simulink model "sampleModel81"  (R2021b)
settings: Solver=VariableStepAuto  StartTime=0.0  StopTime=10.0  RelTol=1e-3
undefined symbols (not defined in the file or in its folder): DiscIntNeverNeededParam
libraries: simulink x9, slpidlib x2
settings Model: Creator=user  LastModifiedBy=user

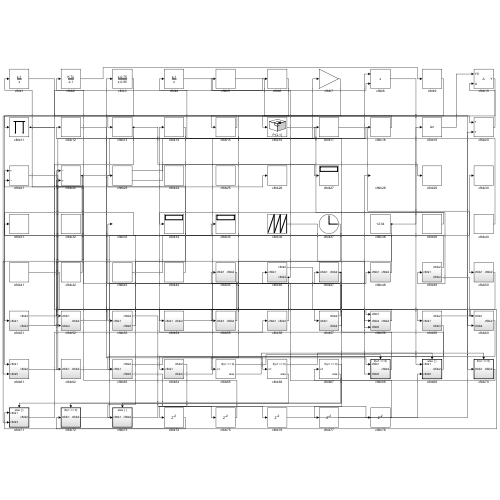
[thumbnail: Simulink's stored preview of the top-level diagram]
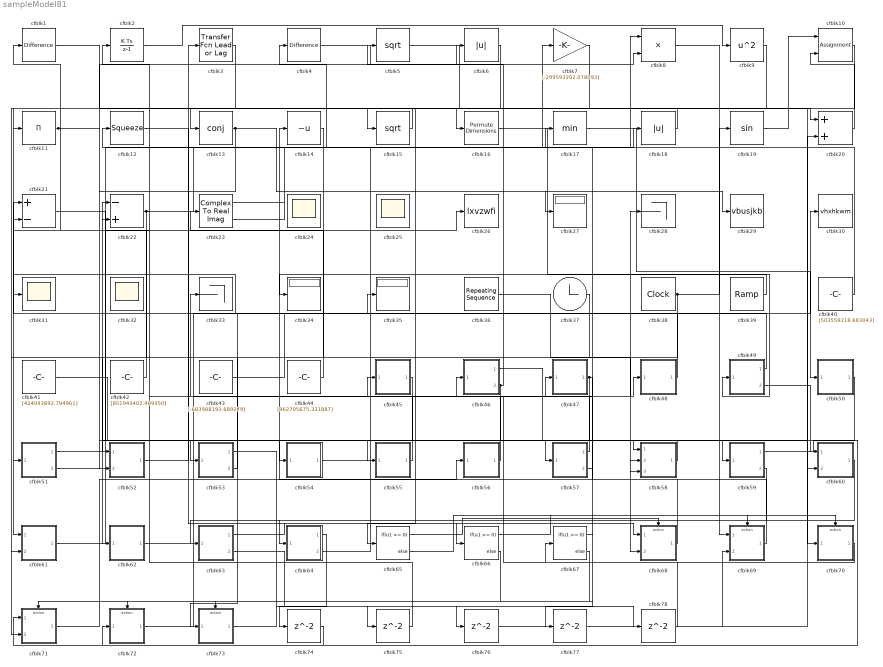
== system sampleModel81 ==
  cfblk1 : simulink/Discrete/Difference  ICPrevInput=0.0  OutMin=[]  OutMax=[]  OutDataTypeStr=Inherit: Inherit via back propagation  OutDataType=fixdt(1, 16)  OutScaling=2^-10  DoSatur=off
  cfblk10 : Assignment  DiagnosticForDimensions=Warning  IndexOptions=Index vector (dialog)  Indices=1  OutputSizes=1
  cfblk11 : Product  Inputs=*
  cfblk12 : Squeeze
  cfblk13 : Math  Operator=conj  SaturateOnIntegerOverflow=on
  cfblk14 : UnaryMinus
  cfblk15 : Sqrt  SaturateOnIntegerOverflow=on
  cfblk16 : PermuteDimensions
  cfblk17 : MinMax
  cfblk18 : Abs
  cfblk19 : Trigonometry
  cfblk2 : DiscreteIntegrator  ICPrevOutput=DiscIntNeverNeededParam  ICPrevScaledInput=DiscIntNeverNeededParam
  cfblk20 : Sum
  cfblk21 : Sum  Inputs=+-
  cfblk22 : Sum  Inputs=-+
  cfblk23 : ComplexToRealImag
  cfblk{24..25,31..32} (4 alike) : Scope
      cfblk24 settings: Floating=on
      cfblk25 settings: Floating=on
      cfblk32 settings: Floating=on
  cfblk26 : ToWorkspace  VariableName=lxvzwfi  SaveFormat=Timeseries  SampleTime=-1
  cfblk27 : Display
  cfblk28 : Terminator
  cfblk29 : ToWorkspace  VariableName=vbusjkb  SaveFormat=Timeseries  SampleTime=-1
  cfblk3 : simulink/Discrete/Transfer Fcn Lead or Lag  PoleZ=0.95  ZeroZ=0.75  ICPrevOutput=0.0  ICPrevInput=0.0  DoSatur=off
      settings: SourceProductBaseCode=SL
  cfblk30 : ToWorkspace  VariableName=vhxhkwm  SaveFormat=Timeseries  SampleTime=-1
  cfblk33 : Terminator
  cfblk34 : Display
  cfblk35 : Display
  cfblk36 : simulink/Sources/Repeating Sequence  rep_seq_t=[0 2]  rep_seq_y=[7788127.978468, 363612122.173200]
  cfblk37 : Clock
  cfblk38 : DigitalClock
  cfblk39 : simulink/Sources/Ramp  slope=[-4423.881026]  start=[41.210749]  InitialOutput=[995796.420869]
  cfblk4 : simulink/Discrete/Difference  ICPrevInput=0.0  OutMin=[]  OutMax=[]  OutDataTypeStr=Inherit: Inherit via back propagation  OutDataType=fixdt(1, 16)  OutScaling=2^-10  DoSatur=off
  cfblk40 : Constant  Value=[503559218.683043]  SampleTime=1
  cfblk41 : Constant  Value=[424093892.794961]  SampleTime=1
  cfblk42 : Constant  Value=[851943402.489350]  SampleTime=1
  cfblk43 : Constant  Value=[-683988193.689279]  SampleTime=1
  cfblk44 : Constant  Value=[962705675.331887]  SampleTime=1
  cfblk45 : Subsystem
  cfblk46 : Subsystem
  cfblk47 : Subsystem
  cfblk48 : Subsystem
  cfblk49 : Subsystem
  cfblk5 : Sqrt  SaturateOnIntegerOverflow=on
  cfblk50 : Subsystem
  cfblk51 : Subsystem
  cfblk52 : Subsystem
  cfblk53 : Subsystem
  cfblk54 : Subsystem
  cfblk55 : Subsystem
  cfblk56 : Subsystem
  cfblk57 : Subsystem
  cfblk58 : Subsystem
  cfblk59 : Subsystem
  cfblk6 : Abs
  cfblk60 : Subsystem
  cfblk61 : Subsystem
  cfblk62 : Subsystem
  cfblk63 : Subsystem
  cfblk64 : Subsystem
  cfblk65 : If  IfExpression=u1 >= 0  SampleTime=1
  cfblk66 : If  IfExpression=u1 >= 0  SampleTime=1
  cfblk67 : If  IfExpression=u1 >= 0  SampleTime=1
  cfblk68 : Subsystem  TreatAsAtomicUnit=on
  cfblk69 : Subsystem  TreatAsAtomicUnit=on
  cfblk7 : Gain  Gain=[-299593202.078093]
  cfblk70 : Subsystem  TreatAsAtomicUnit=on
  cfblk71 : Subsystem  TreatAsAtomicUnit=on
  cfblk72 : Subsystem  TreatAsAtomicUnit=on
  cfblk73 : Subsystem  TreatAsAtomicUnit=on
  cfblk{74..78} (5 alike) : Delay  SampleTime=1
  cfblk8 : Product  Inputs=**
  cfblk9 : Math  Operator=square  SaturateOnIntegerOverflow=on
  wires:
  cfblk60/1(cfblk2) -> cfblk64/1(cfblk1)
  cfblk19/1 -> cfblk10/1
  cfblk47/1(cfblk2) -> cfblk57/1(cfblk1), cfblk77/1
  cfblk69/1(cfblk2) -> cfblk47/1(cfblk1)
  cfblk57/1(cfblk2) -> cfblk33/1
  cfblk49/1(cfblk2) -> cfblk61/1(cfblk1)
  cfblk16/1 -> cfblk49/1(cfblk1)
  cfblk10/1 -> cfblk51/1(cfblk1)
  cfblk20/1 -> cfblk10/2
  cfblk17/1 -> cfblk50/1(cfblk1)
  cfblk64/2(cfblk4) -> cfblk17/1
  cfblk59/1(cfblk2) -> cfblk71/1(cfblk1)
  cfblk62/1(cfblk2) -> cfblk30/1
  cfblk71/1(cfblk2) -> cfblk56/1(cfblk1)
  cfblk68/1(cfblk2) -> cfblk14/1
  cfblk49/2(cfblk4) -> cfblk60/1(cfblk1)
  cfblk57/2(cfblk4) -> cfblk12/1
  cfblk23/1 -> cfblk27/1
  cfblk13/1 -> cfblk29/1, cfblk52/2(cfblk4)
  cfblk72/1(cfblk2) -> cfblk48/1(cfblk1)
  cfblk70/1(cfblk2) -> cfblk67/1
  cfblk39/1 -> cfblk34/1
  cfblk56/1(cfblk2) -> cfblk45/1(cfblk1)
  cfblk6/1 -> cfblk65/1
  cfblk18/1 -> cfblk13/1
  cfblk46/1(cfblk2) -> cfblk59/1(cfblk1)
  cfblk22/1 -> cfblk18/1, cfblk52/1(cfblk1), cfblk21/2
  cfblk38/1 -> cfblk19/1, cfblk55/1(cfblk1)
  cfblk63/1(cfblk2) -> cfblk68/1(cfblk1)
  cfblk12/1 -> cfblk66/1
  cfblk7/1 -> cfblk16/1
  cfblk37/1 -> cfblk71/2(cfblk3)
  cfblk59/2(cfblk3) -> cfblk63/1(cfblk1)
  cfblk21/1 -> cfblk60/2(cfblk4)
  cfblk52/1(cfblk2) -> cfblk3/1
  cfblk43/1 -> cfblk35/1
  cfblk45/1(cfblk2) -> cfblk54/1(cfblk1)
  cfblk50/1(cfblk2) -> cfblk58/1(cfblk1)
  cfblk9/1 -> cfblk15/1
  cfblk61/1(cfblk2) -> cfblk8/1
  cfblk51/1(cfblk2) -> cfblk22/1
  cfblk48/1(cfblk2) -> cfblk21/1
  cfblk58/1(cfblk2) -> cfblk53/1(cfblk1)
  cfblk11/1 -> cfblk58/2(cfblk4), cfblk6/1
  cfblk8/1 -> cfblk69/1(cfblk1)
  cfblk2/1 -> cfblk9/1
  cfblk14/1 -> cfblk73/1(cfblk1)
  cfblk54/1(cfblk2) -> cfblk28/1
  cfblk23/2 -> cfblk7/1
  cfblk41/1 -> cfblk58/3(cfblk5)
  cfblk15/1 -> cfblk11/1
  cfblk3/1 -> cfblk61/2(cfblk5)
  cfblk55/1(cfblk2) -> cfblk2/1
  cfblk36/1 -> cfblk68/2(cfblk5)
  cfblk40/1 -> cfblk4/1
  cfblk53/2(cfblk5) -> cfblk31/1
  cfblk44/1 -> cfblk23/1
  cfblk4/1 -> cfblk8/2
  cfblk42/1 -> cfblk1/1
  cfblk5/1 -> cfblk70/1(cfblk1)
  cfblk1/1 -> cfblk20/1
  cfblk51/2(cfblk3) -> cfblk26/1
  cfblk46/2(cfblk4) -> cfblk62/1(cfblk1), cfblk5/1
  cfblk65/1 -> cfblk68/Action
  cfblk65/2 -> cfblk69/Action
  cfblk66/1 -> cfblk70/Action
  cfblk66/2 -> cfblk71/Action
  cfblk67/1 -> cfblk72/Action
  cfblk67/2 -> cfblk73/Action
  cfblk64/1(cfblk2) -> cfblk74/1
  cfblk74/1 -> cfblk72/1(cfblk1)
  cfblk53/1(cfblk2) -> cfblk75/1
  cfblk75/1 -> cfblk22/2
  cfblk73/1(cfblk2) -> cfblk76/1
  cfblk76/1 -> cfblk69/2(cfblk5)
  cfblk77/1 -> cfblk20/2
  cfblk63/2(cfblk5) -> cfblk78/1
  cfblk78/1 -> cfblk46/1(cfblk1)

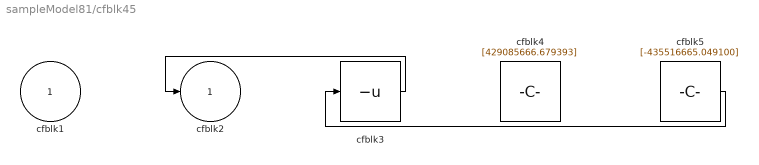
== system sampleModel81/cfblk45 ==
  cfblk1 : Inport
  cfblk3 : UnaryMinus
  cfblk4 : Constant  Value=[429085666.679393]  SampleTime=1
  cfblk5 : Constant  Value=[-435516665.049100]  SampleTime=1
  cfblk2 : Outport
  wires:
  cfblk3/1 -> cfblk2/1
  cfblk5/1 -> cfblk3/1

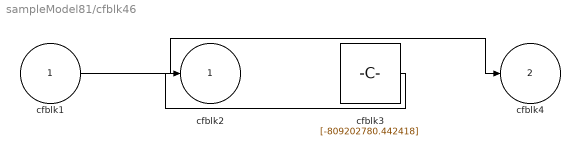
== system sampleModel81/cfblk46 ==
  cfblk1 : Inport
  cfblk3 : Constant  Value=[-809202780.442418]  SampleTime=1
  cfblk2 : Outport
  cfblk4 : Outport  Port=2
  wires:
  cfblk1/1 -> cfblk4/1
  cfblk3/1 -> cfblk2/1

== system sampleModel81/cfblk47 ==
  cfblk1 : Inport
  cfblk3 : DiscreteIntegrator  ICPrevOutput=DiscIntNeverNeededParam  ICPrevScaledInput=DiscIntNeverNeededParam
  cfblk2 : Outport
  wires:
  cfblk3/1 -> cfblk2/1
  cfblk1/1 -> cfblk3/1

== system sampleModel81/cfblk48 ==
  cfblk1 : Inport
  cfblk3 : DiscreteFilter  SampleTime=1
  cfblk2 : Outport
  wires:
  cfblk3/1 -> cfblk2/1
  cfblk1/1 -> cfblk3/1

== system sampleModel81/cfblk49 ==
  cfblk1 : Inport
  cfblk3 : Assignment  DiagnosticForDimensions=Warning  IndexOptions=Index vector (dialog)  Indices=1  OutputSizes=1
  cfblk2 : Outport
  cfblk4 : Outport  Port=2
  wires:
  cfblk1/1 -> cfblk3/1, cfblk2/1, cfblk3/2
  cfblk3/1 -> cfblk4/1

== system sampleModel81/cfblk50 ==
  cfblk1 : Inport
  cfblk3 : Constant  Value=[109728072.236227]  SampleTime=1
  cfblk2 : Outport
  wires:
  cfblk1/1 -> cfblk2/1

== system sampleModel81/cfblk51 ==
  cfblk1 : Inport
  cfblk2 : Outport
  cfblk3 : Outport  Port=2
  wires:
  cfblk1/1 -> cfblk3/1, cfblk2/1

== system sampleModel81/cfblk52 ==
  cfblk1 : Inport
  cfblk4 : Inport  Port=2
  cfblk3 : simulink/Discrete/Difference  ICPrevInput=0.0  OutMin=[]  OutMax=[]  OutDataTypeStr=Inherit: Inherit via back propagation  OutDataType=fixdt(1, 16)  OutScaling=2^-10  DoSatur=off
  cfblk2 : Outport
  wires:
  cfblk1/1 -> cfblk3/1
  cfblk3/1 -> cfblk2/1

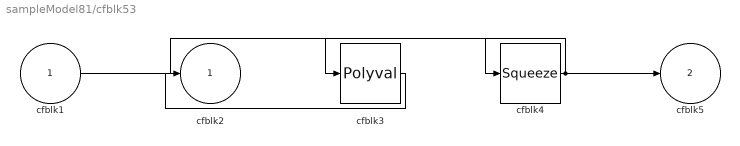
== system sampleModel81/cfblk53 ==
  cfblk1 : Inport
  cfblk3 : Polyval  Coefs=[ +2.081618890e-019, -1.441693666e-014, +4.719686976e-010, -8.536869453e-006, +1.621573104e-001, -8.087801117e+001 ]
  cfblk4 : Squeeze
  cfblk2 : Outport
  cfblk5 : Outport  Port=2
  wires:
  cfblk1/1 -> cfblk4/1
  cfblk3/1 -> cfblk2/1
  cfblk4/1 -> cfblk5/1, cfblk3/1

== system sampleModel81/cfblk54 ==
  cfblk1 : Inport
  cfblk3 : DiscreteZeroPole  Poles=[0 0.5]  Gain=1
  cfblk2 : Outport
  wires:
  cfblk1/1 -> cfblk3/1
  cfblk3/1 -> cfblk2/1

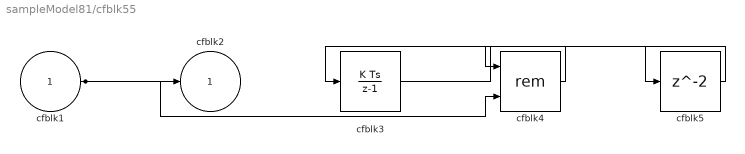
== system sampleModel81/cfblk55 ==
  cfblk1 : Inport
  cfblk3 : DiscreteIntegrator  ICPrevOutput=DiscIntNeverNeededParam  ICPrevScaledInput=DiscIntNeverNeededParam
  cfblk4 : Math  Operator=rem  SaturateOnIntegerOverflow=on
  cfblk5 : Delay  SampleTime=1
  cfblk2 : Outport
  wires:
  cfblk4/1 -> cfblk3/1
  cfblk1/1 -> cfblk2/1, cfblk4/2
  cfblk3/1 -> cfblk5/1
  cfblk5/1 -> cfblk4/1

== system sampleModel81/cfblk56 ==
  cfblk1 : Inport
  cfblk3 : Gain  Gain=[278476586.506630]
  cfblk2 : Outport
  wires:
  cfblk1/1 -> cfblk2/1, cfblk3/1

== system sampleModel81/cfblk57 ==
  cfblk1 : Inport
  cfblk3 : simulink/Math Operations/Slider Gain  gain=1  low=0  high=2
  cfblk2 : Outport
  cfblk4 : Outport  Port=2
  wires:
  cfblk3/1 -> cfblk4/1
  cfblk1/1 -> cfblk2/1, cfblk3/1

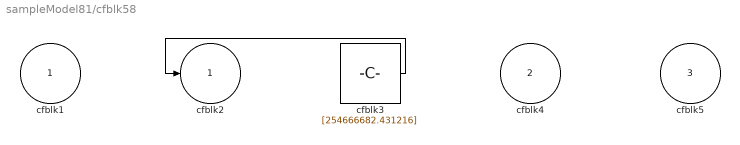
== system sampleModel81/cfblk58 ==
  cfblk1 : Inport
  cfblk4 : Inport  Port=2
  cfblk5 : Inport  Port=3
  cfblk3 : Constant  Value=[254666682.431216]  SampleTime=1
  cfblk2 : Outport
  wires:
  cfblk3/1 -> cfblk2/1

== system sampleModel81/cfblk59 ==
  cfblk1 : Inport
  cfblk2 : Outport
  cfblk3 : Outport  Port=2
  wires:
  cfblk1/1 -> cfblk2/1, cfblk3/1

== system sampleModel81/cfblk60 ==
  cfblk1 : Inport
  cfblk4 : Inport  Port=2
  cfblk3 : Sin  TimeSource=Use external signal  SampleTime=0
  cfblk2 : Outport
  wires:
  cfblk1/1 -> cfblk2/1
  cfblk4/1 -> cfblk3/1

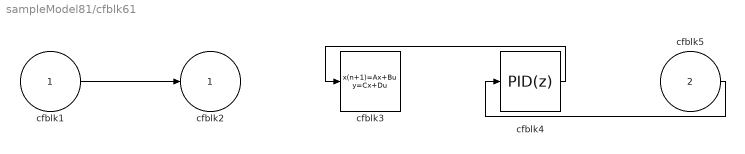
== system sampleModel81/cfblk61 ==
  cfblk1 : Inport
  cfblk5 : Inport  Port=2
  cfblk3 : DiscreteStateSpace
  cfblk4 : slpidlib/PID Controller  Controller=PID  Form=Parallel  TimeDomain=Discrete-time  UseExternalTs=off  SampleTime=1  IntegratorMethod=Forward Euler  FilterMethod=Forward Euler  ControllerParametersSource=internal  P=1  I=1  D=0  UseFilter=on  N=100  TunerSelectOption=Transfer Function Based (PID Tuner App)  InitialConditionSource=internal  InitialConditionForIntegrator=0  InitialConditionForFilter=0  DifferentiatorICPrevScaledInput=0  ExternalReset=none  TrackingMode=off  Kt=1  LimitOutput=off  SatLimitsSource=internal  UpperSaturationLimit=inf  LowerSaturationLimit=-inf  LinearizeAsGain=off  AntiWindupMode=none  Kb=1  POutMin=[]  POutMax=[]  IOutMin=[]  IOutMax=[]  DOutMin=[]  DOutMax=[]  NOutMin=[]  NOutMax=[]  SumOutMin=[]  SumOutMax=[]  SaturationOutMin=[]  SaturationOutMax=[]  PParamMin=[]  PParamMax=[]  IParamMin=[]  IParamMax=[]  DParamMin=[]  DParamMax=[]  NParamMin=[]  NParamMax=[]  KbParamMin=[]  KbParamMax=[]  KtParamMin=[]  KtParamMax=[]  KbOutMin=[]  KbOutMax=[]  KtOutMin=[]  KtOutMax=[]  IntegratorOutMin=[]  IntegratorOutMax=[]  FilterOutMin=[]  FilterOutMax=[]  SumI1OutMin=[]  SumI1OutMax=[]  SumI2OutMin=[]  SumI2OutMax=[]  SumI3OutMin=[]  SumI3OutMax=[]  SumI4OutMin=[]  SumI4OutMax=[]  SumDOutMin=[]  SumDOutMax=[]  DifferentiatorOutMin=[]  DifferentiatorOutMax=[]  FilterDiffOutCoefMin=[]  FilterDiffOutCoefMax=[]  ReciprocalOutMin=[]  ReciprocalOutMax=[]  SumDenOutMin=[]  SumDenOutMax=[]  SumNumOutMin=[]  SumNumOutMax=[]  DivideOutMin=[]  DivideOutMax=[]  UdiffTsProdOutMin=[]  UdiffTsProdOutMax=[]  NTsProdOutMin=[]  NTsProdOutMax=[]  UintegralTsProdOutMin=[]  UintegralTsProdOutMax=[]  UngainTsProdOutMin=[]  UngainTsProdOutMax=[]  IntegratorContinuousStateAttributes=''  IntegratorStateMustResolveToSignalObject=off  IntegratorRTWStateStorageClass=Auto  FilterContinuousStateAttributes=''  FilterStateMustResolveToSignalObject=off  FilterRTWStateStorageClass=Auto  ParallelPVariant=InternalParameters  IdealPVariant=Disabled  IVariant=InternalParameters  DVariant=InternalParameters  IntegratorVariant=Discrete  SatVariant=Disabled  AWVariant=Passthrough  PCopyVariant=Disabled  TRVariant=Disabled  FdbkBlocksVariant=Forward  IdealPFdbkVariant=Disabled  SatFdbkVariant=Disabled  DerivativeFilterVariant=ForwardEulerFilter  NVariant=InternalParameters  NCopyVariant=Disabled  FilterICVariant=InternalICsFilter  IntegratorICVariant=InternalICs  ExternalResetVariant=Disabled  TRSumVariant=Passthrough  SumFdbkVariant=Disabled  SumVariant=Sum_PID  TsampFilterVariant=InternalTs  TsampNgainVariant=Passthrough  TsampIntegralVariant=Passthrough  ExternalSaturationOutDataTypeStr=Inherit: Same as second input
  cfblk2 : Outport
  wires:
  cfblk4/1 -> cfblk3/1
  cfblk1/1 -> cfblk2/1
  cfblk5/1 -> cfblk4/1

== system sampleModel81/cfblk62 ==
  cfblk1 : Inport
  cfblk3 : simulink/Discrete/Difference  ICPrevInput=0.0  OutMin=[]  OutMax=[]  OutDataTypeStr=Inherit: Inherit via back propagation  OutDataType=fixdt(1, 16)  OutScaling=2^-10  DoSatur=off
  cfblk4 : ComplexToRealImag
  cfblk2 : Outport
  wires:
  cfblk1/1 -> cfblk4/1
  cfblk4/1 -> cfblk3/1
  cfblk3/1 -> cfblk2/1

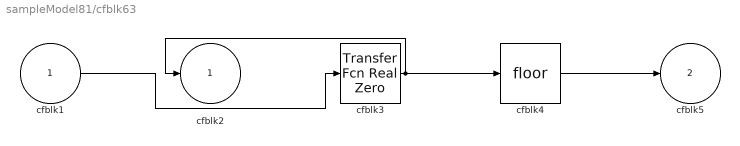
== system sampleModel81/cfblk63 ==
  cfblk1 : Inport
  cfblk3 : simulink/Discrete/Transfer Fcn Real Zero  ZeroZ=0.75  ICPrevInput=0.0  DoSatur=off
      settings: SourceProductBaseCode=SL
  cfblk4 : Rounding
  cfblk2 : Outport
  cfblk5 : Outport  Port=2
  wires:
  cfblk3/1 -> cfblk2/1, cfblk4/1
  cfblk1/1 -> cfblk3/1
  cfblk4/1 -> cfblk5/1

== system sampleModel81/cfblk64 ==
  cfblk1 : Inport
  cfblk3 : slpidlib/PID Controller  Controller=PID  Form=Parallel  TimeDomain=Discrete-time  UseExternalTs=off  SampleTime=1  IntegratorMethod=Forward Euler  FilterMethod=Forward Euler  ControllerParametersSource=internal  P=1  I=1  D=0  UseFilter=on  N=100  TunerSelectOption=Transfer Function Based (PID Tuner App)  InitialConditionSource=internal  InitialConditionForIntegrator=0  InitialConditionForFilter=0  DifferentiatorICPrevScaledInput=0  ExternalReset=none  TrackingMode=off  Kt=1  LimitOutput=off  SatLimitsSource=internal  UpperSaturationLimit=inf  LowerSaturationLimit=-inf  LinearizeAsGain=off  AntiWindupMode=none  Kb=1  POutMin=[]  POutMax=[]  IOutMin=[]  IOutMax=[]  DOutMin=[]  DOutMax=[]  NOutMin=[]  NOutMax=[]  SumOutMin=[]  SumOutMax=[]  SaturationOutMin=[]  SaturationOutMax=[]  PParamMin=[]  PParamMax=[]  IParamMin=[]  IParamMax=[]  DParamMin=[]  DParamMax=[]  NParamMin=[]  NParamMax=[]  KbParamMin=[]  KbParamMax=[]  KtParamMin=[]  KtParamMax=[]  KbOutMin=[]  KbOutMax=[]  KtOutMin=[]  KtOutMax=[]  IntegratorOutMin=[]  IntegratorOutMax=[]  FilterOutMin=[]  FilterOutMax=[]  SumI1OutMin=[]  SumI1OutMax=[]  SumI2OutMin=[]  SumI2OutMax=[]  SumI3OutMin=[]  SumI3OutMax=[]  SumI4OutMin=[]  SumI4OutMax=[]  SumDOutMin=[]  SumDOutMax=[]  DifferentiatorOutMin=[]  DifferentiatorOutMax=[]  FilterDiffOutCoefMin=[]  FilterDiffOutCoefMax=[]  ReciprocalOutMin=[]  ReciprocalOutMax=[]  SumDenOutMin=[]  SumDenOutMax=[]  SumNumOutMin=[]  SumNumOutMax=[]  DivideOutMin=[]  DivideOutMax=[]  UdiffTsProdOutMin=[]  UdiffTsProdOutMax=[]  NTsProdOutMin=[]  NTsProdOutMax=[]  UintegralTsProdOutMin=[]  UintegralTsProdOutMax=[]  UngainTsProdOutMin=[]  UngainTsProdOutMax=[]  IntegratorContinuousStateAttributes=''  IntegratorStateMustResolveToSignalObject=off  IntegratorRTWStateStorageClass=Auto  FilterContinuousStateAttributes=''  FilterStateMustResolveToSignalObject=off  FilterRTWStateStorageClass=Auto  ParallelPVariant=InternalParameters  IdealPVariant=Disabled  IVariant=InternalParameters  DVariant=InternalParameters  IntegratorVariant=Discrete  SatVariant=Disabled  AWVariant=Passthrough  PCopyVariant=Disabled  TRVariant=Disabled  FdbkBlocksVariant=Forward  IdealPFdbkVariant=Disabled  SatFdbkVariant=Disabled  DerivativeFilterVariant=ForwardEulerFilter  NVariant=InternalParameters  NCopyVariant=Disabled  FilterICVariant=InternalICsFilter  IntegratorICVariant=InternalICs  ExternalResetVariant=Disabled  TRSumVariant=Passthrough  SumFdbkVariant=Disabled  SumVariant=Sum_PID  TsampFilterVariant=InternalTs  TsampNgainVariant=Passthrough  TsampIntegralVariant=Passthrough  ExternalSaturationOutDataTypeStr=Inherit: Same as second input
  cfblk2 : Outport
  cfblk4 : Outport  Port=2
  wires:
  cfblk1/1 -> cfblk2/1, cfblk3/1
  cfblk3/1 -> cfblk4/1

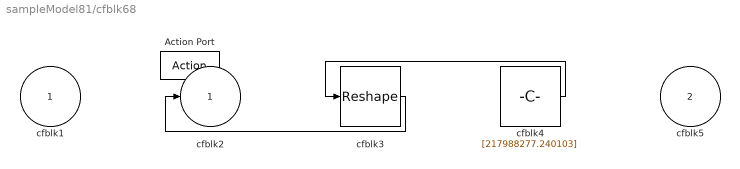
== system sampleModel81/cfblk68 ==
  cfblk1 : Inport
  cfblk5 : Inport  Port=2
  Action Port : ActionPort  ActionPortLabel=if(u1 >= 0)
  cfblk3 : Reshape
  cfblk4 : Constant  Value=[217988277.240103]  SampleTime=1
  cfblk2 : Outport
  wires:
  cfblk3/1 -> cfblk2/1
  cfblk4/1 -> cfblk3/1

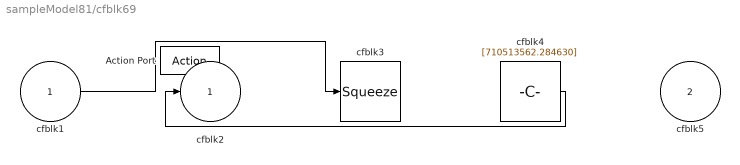
== system sampleModel81/cfblk69 ==
  cfblk1 : Inport
  cfblk5 : Inport  Port=2
  Action Port : ActionPort  ActionPortLabel=else
  cfblk3 : Squeeze
  cfblk4 : Constant  Value=[710513562.284630]  SampleTime=1
  cfblk2 : Outport
  wires:
  cfblk4/1 -> cfblk2/1
  cfblk1/1 -> cfblk3/1

== system sampleModel81/cfblk70 ==
  cfblk1 : Inport
  Action Port : ActionPort  ActionPortLabel=if(u1 >= 0)
  cfblk3 : Sqrt  SaturateOnIntegerOverflow=on
  cfblk2 : Outport
  wires:
  cfblk1/1 -> cfblk3/1
  cfblk3/1 -> cfblk2/1

== system sampleModel81/cfblk71 ==
  cfblk1 : Inport
  cfblk3 : Inport  Port=2
  Action Port : ActionPort  ActionPortLabel=else
  cfblk2 : Outport
  wires:
  cfblk3/1 -> cfblk2/1

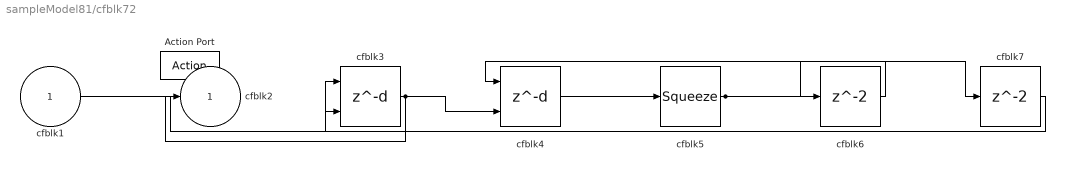
== system sampleModel81/cfblk72 ==
  cfblk1 : Inport
  Action Port : ActionPort  ActionPortLabel=if(u1 >= 0)
  cfblk3 : Delay  DelayLengthSource=Input port
      settings: InputPortMap=u0,p1
  cfblk4 : Delay  DelayLengthSource=Input port
      settings: InputPortMap=u0,p1
  cfblk5 : Squeeze
  cfblk6 : Delay
  cfblk7 : Delay
  cfblk2 : Outport
  wires:
  cfblk4/1 -> cfblk5/1
  cfblk1/1 -> cfblk3/1
  cfblk5/1 -> cfblk6/1, cfblk7/1
  cfblk3/1 -> cfblk2/1, cfblk4/2
  cfblk6/1 -> cfblk4/1
  cfblk7/1 -> cfblk3/2

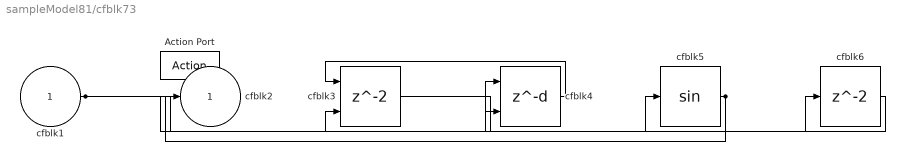
== system sampleModel81/cfblk73 ==
  cfblk1 : Inport
  Action Port : ActionPort  ActionPortLabel=else
  cfblk3 : Delay  ShowEnablePort=on
      settings: InputPortMap=u0,e6
  cfblk4 : Delay  DelayLengthSource=Input port
      settings: InputPortMap=u0,p1
  cfblk5 : Trigonometry
  cfblk6 : Delay
  cfblk2 : Outport
  wires:
  cfblk1/1 -> cfblk4/1, cfblk5/1
  cfblk5/1 -> cfblk2/1, cfblk3/2
  cfblk4/1 -> cfblk3/1
  cfblk3/1 -> cfblk6/1
  cfblk6/1 -> cfblk4/2
